simulink model "mfc_mod"  (Simulink 3.00)
settings: Solver=ode45  StartTime=0.0  StopTime=100.0  RelTol=1e-3
values from neighbouring files (symbols this model uses):
  stack = struct('general',[],'evaluation',[],'simulation',[],'temp',[])    [gohome.m]
settings Model: SaveTime=off  SaveOutput=off

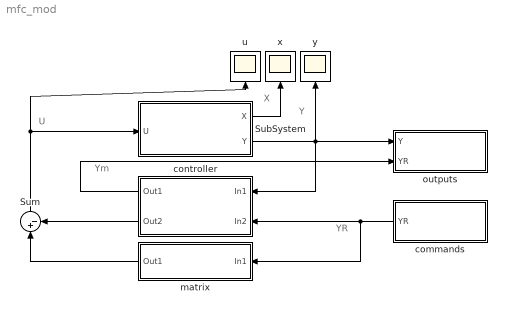
== system mfc_mod ==
  note: U
  note: Y
  note: YR
  note: X
  note: Ym
  SubSystem : Subsystem
      mask Display: disp('PLANT')
  Sum : Sum  Orientation=up  Inputs=|+-  SaturateOnIntegerOverflow=on
  commands : Subsystem  Orientation=left
      mask Display: disp('COMMANDS')
  controller : Subsystem  Orientation=left
      mask Display: disp('CONTROLLER')
  matrix : Subsystem  Orientation=left
      mask Display: disp('Kpf')
  outputs : Subsystem
      mask Display: disp('OUTPUTS')
  u : Scope
      settings: Orientation=up  TimeRange=auto  YMin=-5  YMax=5  SaveToWorkspace=off  SaveName=ScopeData
  x : Scope
      settings: Orientation=up  TimeRange=auto  YMin=-5  YMax=5  SaveToWorkspace=off  SaveName=ScopeData
  y : Scope
      settings: Orientation=up  TimeRange=auto  YMin=-5  YMax=5  SaveToWorkspace=off  SaveName=ScopeData
  wires:
  matrix/1(Out1) -> Sum/1
  SubSystem/1(X) -> x/1
  Sum/1 -> SubSystem/1(U), u/1
  SubSystem/2(Y) -> outputs/1(Y), y/1, controller/1(In1)
  commands/1(YR) -> matrix/1(In1), controller/2(In2)
  controller/2(Out2) -> Sum/2
  controller/1(Out1) -> outputs/2(YR)

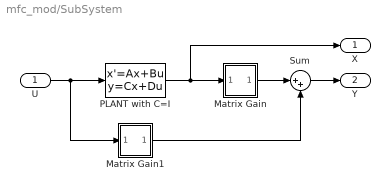
== system mfc_mod/SubSystem ==
  U : Inport  Port=1  PortWidth=-1  SampleTime=-1  DataType=auto
      settings: SignalType=auto
  Matrix Gain : Subsystem  mask(Matrix Gain){K=stack.general.C}
      mask prompts: K "Gain matrix:"
      mask help: Matrix Gain.
      mask Help: Multiplies input vector by entered matrix to produce output vector (y=Au).
      mask Display: disp('C')
  Matrix Gain1 : Subsystem  mask(Matrix Gain){K=stack.general.D}
      mask prompts: K "Gain matrix:"
      mask help: Matrix Gain.
      mask Help: Multiplies input vector by entered matrix to produce output vector (y=Au).
      mask Display: disp('D')
  PLANT with C=I : StateSpace  A=stack.general.A  B=stack.general.B  C=eye(size(stack.general.A))  D=zeros(size(stack.general.A,1),size(stack.general.B,2))  X0=0
  Sum : Sum  Inputs=|++  SaturateOnIntegerOverflow=on
  X : Outport  Port=1
  Y : Outport  Port=2
  wires:
  Matrix Gain/1(Out1) -> Sum/1
  Sum/1 -> Y/1
  PLANT with C=I/1 -> Matrix Gain/1(In1), X/1
  Matrix Gain1/1(Out1) -> Sum/2
  U/1 -> PLANT with C=I/1, Matrix Gain1/1(In1)

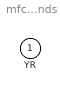
== system mfc_mod/commands ==
  YR : Outport  Orientation=left  Port=1

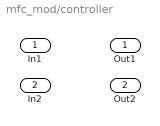
== system mfc_mod/controller ==
  In1 : Inport  Port=1  PortWidth=-1  SampleTime=-1  DataType=auto
      settings: SignalType=auto
  In2 : Inport  Port=2  PortWidth=-1  SampleTime=-1  DataType=auto
      settings: SignalType=auto
  Out1 : Outport  Port=1
  Out2 : Outport  Port=2

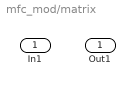
== system mfc_mod/matrix ==
  In1 : Inport  Port=1  PortWidth=-1  SampleTime=-1  DataType=auto
      settings: SignalType=auto
  Out1 : Outport  Port=1

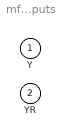
== system mfc_mod/outputs ==
  Y : Inport  Port=1  PortWidth=-1  SampleTime=0  DataType=auto
      settings: SignalType=auto
  YR : Inport  Port=2  PortWidth=-1  SampleTime=0  DataType=auto
      settings: SignalType=auto

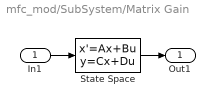
== system mfc_mod/SubSystem/Matrix Gain ==
  In1 : Inport  Port=1  PortWidth=-1  SampleTime=-1  DataType=auto
      settings: SignalType=auto
  State Space : StateSpace  A=[]  B=[]  C=[]  D=K  X0=0
  Out1 : Outport  Port=1
  wires:
  In1/1 -> State Space/1
  State Space/1 -> Out1/1

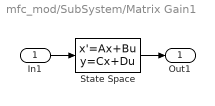
== system mfc_mod/SubSystem/Matrix Gain1 ==
  In1 : Inport  Port=1  PortWidth=-1  SampleTime=-1  DataType=auto
      settings: SignalType=auto
  State Space : StateSpace  A=[]  B=[]  C=[]  D=K  X0=0
  Out1 : Outport  Port=1
  wires:
  In1/1 -> State Space/1
  State Space/1 -> Out1/1
